simulink model "lr2"  (R2024a)
settings: Solver=ode23tb  StartTime=0.0  StopTime=0.4  MaxStep=2e-4  RelTol=1e-4
undefined symbols (not defined in the file or in its folder): control, load, source, transparam
libraries: spsFourierLib x4, spsGroundLib x4, spsCurrentMeasurementLib x3, spsVoltageMeasurementLib x2, spsACVoltageSourceLib x1, spsDCVoltageSourceLib x1, spsDiodeLib x1, spsLinearTransformerLib x1, spsMultimeterLib x1, spsRMSLib x1, spsSeriesRLCBranchLib x1, spsUniversalBridgeLib x1
settings Model: Creator=Руслан  LastModifiedBy=79532
settings SolverCC: SolverResetMethod=Robust
settings OptimizationCC: ReuseModelBlockBuffer=off
settings RTWCC: GPUComputeCapability=3.5

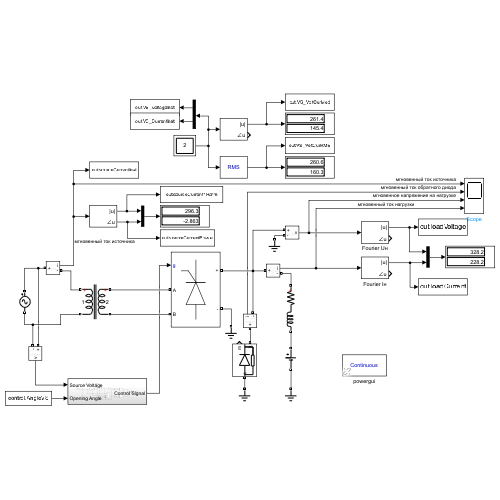
[thumbnail: Simulink's stored preview of the top-level diagram]
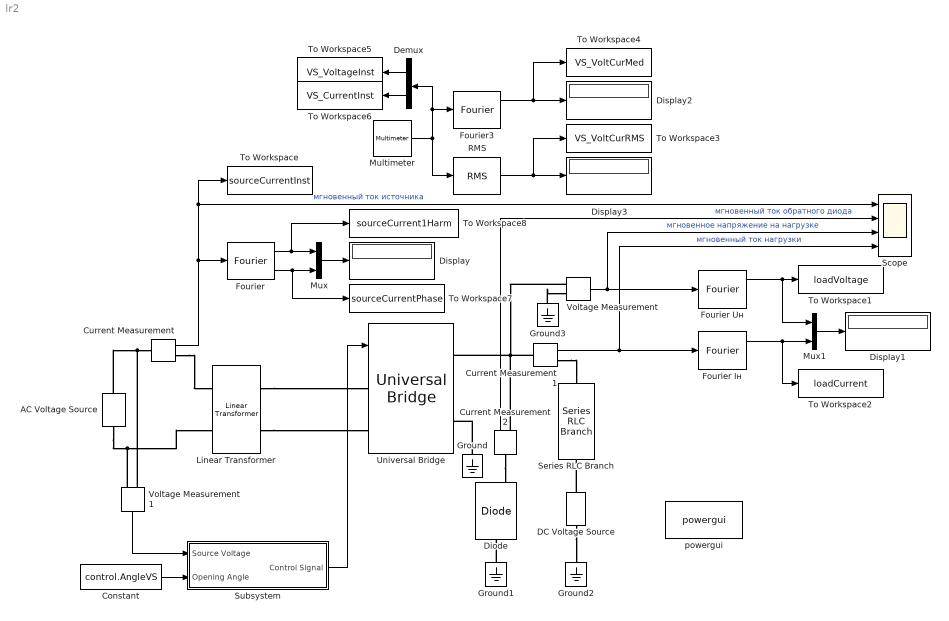
== system lr2 ==
  AC Voltage Source : spsACVoltageSourceLib/AC Voltage Source  Amplitude=source.voltageMag  Phase=0  Frequency=source.freq  SampleTime=0  Measurements=None  BusType=swing  Pref=10e3  Qref=0  Qmin=-inf  Qmax=+inf
  Constant : Constant  Value=control.AngleVS
  Current Measurement : spsCurrentMeasurementLib/Current Measurement  PhasorSimulation=off  OutputType=Complex  PSBequivalent=0
  Current Measurement1 : spsCurrentMeasurementLib/Current Measurement  PhasorSimulation=off  OutputType=Complex  PSBequivalent=0
  Current Measurement2 : spsCurrentMeasurementLib/Current Measurement  PhasorSimulation=off  OutputType=Complex  PSBequivalent=0
  DC Voltage Source : spsDCVoltageSourceLib/DC Voltage Source  Amplitude=load.EMF  Measurements=None
  Demux : Demux  Outputs=2
  Diode : spsDiodeLib/Diode  Ron=0.001  Lon=0  Vf=0.8  IC=0  UseSnubber=0  Rs=500  Cs=250e-9  Measurements=on
  Display{,1..3} (4 alike) : Display
      settings: Decimation=2
  Fourier : spsFourierLib/Fourier  Freq=source.freq  n=1  InInit=[0, 0]  Ts=0
  Fourier Iн : spsFourierLib/Fourier  Freq=source.freq*2  n=0  InInit=[0, 0]  Ts=0
  Fourier Uн : spsFourierLib/Fourier  Freq=source.freq*2  n=0  InInit=[0, 0]  Ts=0
  Fourier3 : spsFourierLib/Fourier  Freq=source.freq  n=1  InInit=[0, 0]  Ts=0
  Ground{,1..3} (4 alike) : spsGroundLib/Ground  LConnTagsString=a
  Linear Transformer : spsLinearTransformerLib/Linear Transformer  UNITS=SI  NominalPower=[ transparam.power source.freq ]  winding1=[transparam.volt1wing 0.01 0.000001]  winding2=[transparam.volt2wing 0.04 0.000004]  ThreeWindings=off  winding3=[3.15e+05 0.7938 0.084225]  RmLm=[100 2]  Measurements=None  DataType=on
  Multimeter : spsMultimeterLib/Multimeter  L=10  sel=[1 7]  yselected={}  Gain=[1 1]  OutputType=Complex  PlotAtSimulationStop=on  PhasorSimulation=off
  Mux : Mux  Inputs=2
  Mux1 : Mux  Inputs=2
  RMS : spsRMSLib/RMS  TrueRMS=on  Freq=source.freq  RMSInit=120  Ts=0
  Scope : Scope  NumInputPorts=4
  Series RLC Branch : spsSeriesRLCBranchLib/Series RLC Branch  LConnTagsString=__new0  RConnTagsString=__new0  BranchType=RL  Resistance=load.Res  Inductance=load.Ind  SetiL0=off  InitialCurrent=0  Capacitance=1e-6  Setx0=off  InitialVoltage=0  Measurements=None
  Subsystem : Subsystem
  To Workspace : ToWorkspace  VariableName=sourceCurrentInst  SampleTime=2e-4
      settings: MaxDataPoints=200  Save2DSignal=2-D array (concatenate along first dimension)
  To Workspace1 : ToWorkspace  VariableName=loadVoltage  SampleTime=2e-4
      settings: MaxDataPoints=200  Save2DSignal=2-D array (concatenate along first dimension)
  To Workspace2 : ToWorkspace  VariableName=loadCurrent  SampleTime=2e-4
      settings: MaxDataPoints=200  Save2DSignal=2-D array (concatenate along first dimension)
  To Workspace3 : ToWorkspace  VariableName=VS_VoltCurRMS  SampleTime=2e-4
      settings: MaxDataPoints=200  Save2DSignal=2-D array (concatenate along first dimension)
  To Workspace4 : ToWorkspace  VariableName=VS_VoltCurMed  SampleTime=2e-4
      settings: MaxDataPoints=200  Save2DSignal=2-D array (concatenate along first dimension)
  To Workspace5 : ToWorkspace  VariableName=VS_VoltageInst  SampleTime=2e-4
      settings: MaxDataPoints=200  Save2DSignal=2-D array (concatenate along first dimension)
  To Workspace6 : ToWorkspace  VariableName=VS_CurrentInst  SampleTime=2e-4
      settings: MaxDataPoints=200  Save2DSignal=2-D array (concatenate along first dimension)
  To Workspace7 : ToWorkspace  VariableName=sourceCurrentPhase  SampleTime=2e-4
      settings: MaxDataPoints=200  Save2DSignal=2-D array (concatenate along first dimension)
  To Workspace8 : ToWorkspace  VariableName=sourceCurrent1Harm  SampleTime=2e-4
      settings: MaxDataPoints=200  Save2DSignal=2-D array (concatenate along first dimension)
  Universal Bridge : spsUniversalBridgeLib/Universal Bridge  Arms=2  SnubberResistance=1e5  SnubberCapacitance=1e-6  Device=Thyristors  Ron=VS.InternalResistance  Lon=0  ForwardVoltages="[  0  0  ]"  ForwardVoltage=VS.ForwardVoltage  GTOparameters=[ 10e-6 , 20e-6 ]  IGBTparameters=[ 1e-6 , 2e-6 ]  Measurements=All voltages and currents  Measurements_2=None  converterType=Rectifier
  Voltage Measurement : spsVoltageMeasurementLib/Voltage Measurement  PhasorSimulation=off  OutputType=Complex  PSBequivalent=0
  Voltage Measurement1 : spsVoltageMeasurementLib/Voltage Measurement  PhasorSimulation=off  OutputType=Complex  PSBequivalent=0
  powergui : sps_lib/powergui  Priority=1  SimulationMode=Continuous  SampleTime=50e-6  frequency=60  Iterations=50  frequencyindice=50  Pbase=100e6  ErrMax=1e-4  UnitsV=kV  UnitsW=MW  buscounter=0  FunctionMessages=off  echomessages=off  EnableUseOfTLC=off  CurrentSourceSwitches=off  DisableSnubberDevices=off  DisableRonSwitches=off  DisableVfSwitches=off  DisplayEquations=off  AutomaticDiscreteSolvers=off  SolverType=Tustin/Backward Euler (TBE)  Interpol=off  ExternalGateDelay=off  methode=off  Ts=100  x0status=blocks  SPID=on  SwTol=0  HookPort=off  NonlinearTolerance=1e-4  nMaxIteration=100  ContinueOnMaxIteration=off  RestoreLinks=warning  ResistiveCurrentMeasurement=off  Frange=[0:2:500]  Ylog=off  Xlog=on  ShowGrid=off  save=off  variable=ZData  structure=0  ZoomFFT=off  StartTime=0.0  cycles=1  DisplayStyle=1  fundamental=60  FreqAxis=off  MaxFrequency=1000  frequencyindicesteady=1  RmsSteady=1  display=off
  wires:
  Current Measurement/1 -> To Workspace/1, Scope/1, Fourier/1  "мгновенный ток источника"
  Multimeter/1 -> RMS/1, Demux/1, Fourier3/1
  Voltage Measurement1/1 -> Subsystem/1(Source Voltage)
  Subsystem/1(Control Signal) -> Universal Bridge/1
  Fourier/1 -> To Workspace8/1, Mux/1
  Fourier/2 -> To Workspace7/1, Mux/2
  Mux/1 -> Display/1
  Current Measurement1/1 -> Scope/4, Fourier Iн/1  "мгновенный ток нагрузки"
  Voltage Measurement/1 -> Scope/3, Fourier Uн/1  "мгновенное напряжение на нагрузке"
  Fourier Uн/1 -> To Workspace1/1, Mux1/1
  Fourier Iн/1 -> To Workspace2/1, Mux1/2
  Mux1/1 -> Display1/1
  Current Measurement2/1 -> Scope/2  "мгновенный ток обратного диода"
  Fourier3/1 -> To Workspace4/1, Display2/1
  RMS/1 -> To Workspace3/1, Display3/1
  Demux/1 -> To Workspace5/1
  Demux/2 -> To Workspace6/1
  Constant/1 -> Subsystem/2(Opening Angle)
  connections:
  AC Voltage Source/RConn1 -- Voltage Measurement1/LConn1 -- Current Measurement/LConn1
  Current Measurement/RConn1 -- Linear Transformer/LConn1
  AC Voltage Source/LConn1 -- Voltage Measurement1/LConn2 -- Linear Transformer/LConn2
  Linear Transformer/RConn1 -- Universal Bridge/LConn1
  Linear Transformer/RConn2 -- Universal Bridge/LConn2
  Current Measurement1/LConn1 -- Universal Bridge/RConn1 -- Voltage Measurement/LConn1 -- Current Measurement2/RConn1
  Current Measurement1/RConn1 -- Series RLC Branch/LConn1
  Ground/LConn1 -- Universal Bridge/RConn2
  Ground1/LConn1 -- Diode/LConn1
  DC Voltage Source/RConn1 -- Series RLC Branch/RConn1
  DC Voltage Source/LConn1 -- Ground2/LConn1
  Current Measurement2/LConn1 -- Diode/RConn1
  Ground3/LConn1 -- Voltage Measurement/LConn2

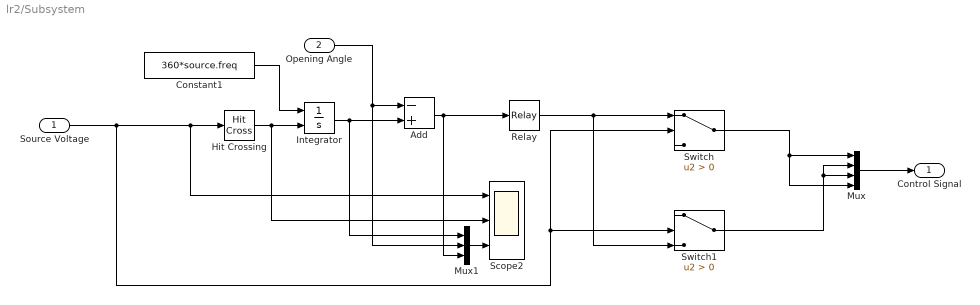
== system lr2/Subsystem ==
  Source Voltage : Inport
  Opening Angle : Inport  Port=2
  Add : Sum  Inputs=-+
  Constant1 : Constant  Value=360*source.freq
  Hit Crossing : HitCross
  Integrator : Integrator  ExternalReset=rising
  Mux : Mux
  Mux1 : Mux  Inputs=3
  Relay : Relay
  Scope2 : Scope  NumInputPorts=3
  Switch : Switch  Criteria=u2 > Threshold  SaturateOnIntegerOverflow=off  InputSameDT=off
  Switch1 : Switch  Criteria=u2 > Threshold  SaturateOnIntegerOverflow=off  InputSameDT=off
  Control Signal : Outport
  wires:
  Relay/1 -> Switch1/3, Switch/1
  Opening Angle/1 -> Add/1, Mux1/2
  Source Voltage/1 -> Switch1/2, Switch/2, Scope2/1, Hit Crossing/1
  Integrator/1 -> Mux1/1, Add/2
  Constant1/1 -> Integrator/1
  Switch/1 -> Mux/1, Mux/4
  Add/1 -> Mux1/3, Relay/1
  Hit Crossing/1 -> Scope2/2, Integrator/2
  Mux1/1 -> Scope2/3
  Switch1/1 -> Mux/3, Mux/2
  Mux/1 -> Control Signal/1
